simulink model "moteur_plus_gene_plus_charge_plus_frottement_22_09_2025"  (R2025b)
settings: Solver=VariableStepAuto  StartTime=0.0  StopTime=0.1  FixedStep=1e-4  RelTol=1e-3
values from neighbouring files (symbols this model uses):
  C0 = 2.4*10^-2    (= 0.024)    [donnee_moteur_seul_22_09_2025.m]
  f = (0.53*30*10^-2)/(1000*pi)    (= 5.06112719032e-05)    [donnee_moteur_seul_22_09_2025.m]
  J = 8.3e-5    (= 8.3e-05)    [donnee_moteur_seul_22_09_2025.m]
  Kphi = 0.127    [donnee_moteur_seul_22_09_2025.m]
  L = 2.2e-3    (= 0.0022)    [donnee_moteur_seul_22_09_2025.m]
  R = 1.52    [donnee_moteur_seul_22_09_2025.m]
  Rch = 10    [donnee_moteur_seul_22_09_2025.m]
  U = 48    [donnee_moteur_seul_22_09_2025.m]
settings Model: Creator=ltroullier01  LastModifiedBy=rudyv

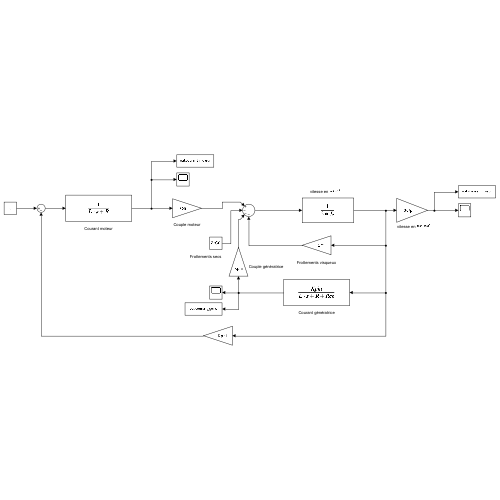
[thumbnail: Simulink's stored preview of the top-level diagram]
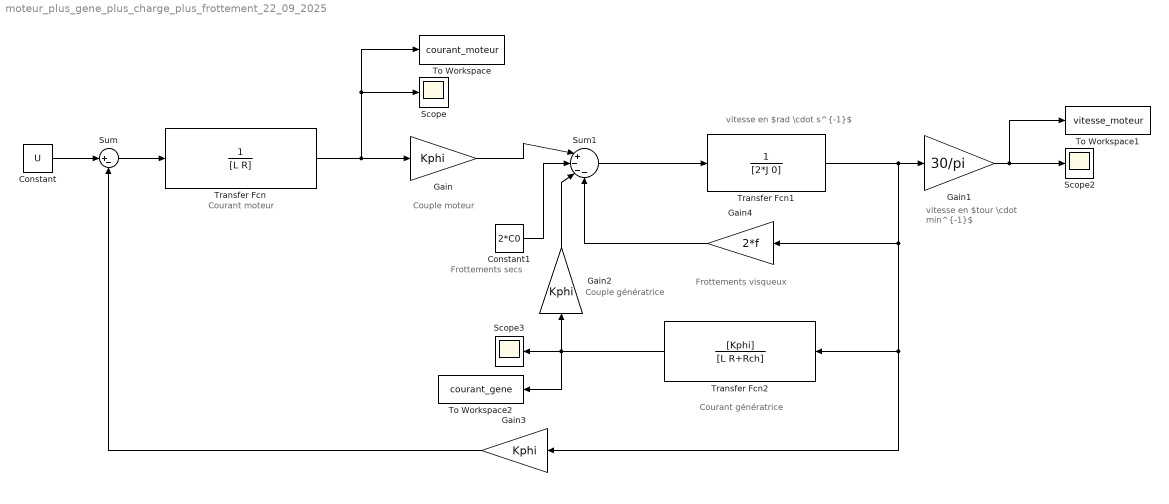
== system moteur_plus_gene_plus_charge_plus_frottement_22_09_2025 ==
  note: Courant génératrice
  note: Couple génératrice
  note: Frottements visqueux
  note: vitesse en $tour \cdot min^{-1}$
  note: Couple moteur
  note: Frottements secs
  note: Courant moteur
  note: vitesse en $rad \cdot s^{-1}$
  Constant : Constant  Value=U
  Constant1 : Constant  Value=2*C0
  Gain : Gain  Gain=Kphi
  Gain1 : Gain  Gain=30/pi
  Gain2 : Gain  Gain=Kphi
  Gain3 : Gain  Gain=Kphi
  Gain4 : Gain  Gain=2*f
  Scope : Scope
      settings: ActiveDisplayYMinimum=-4.9369832712561159  ActiveDisplayYMaximum=31.373841687864346
  Scope2 : Scope
      settings: ActiveDisplayYMinimum=-1903.7496929081253  ActiveDisplayYMaximum=5096.5030674299223  DataLoggingVariableName=ScopeData2
  Scope3 : Scope
      settings: ActiveDisplayYMinimum=-4.9369832712561159  ActiveDisplayYMaximum=31.373841687864346  DataLoggingVariableName=ScopeData3
  Sum : Sum  Inputs=|+-
  Sum1 : Sum  Inputs=|+---
  To Workspace : ToWorkspace  VariableName=courant_moteur  SaveFormat=Timeseries  SampleTime=-1
  To Workspace1 : ToWorkspace  VariableName=vitesse_moteur  SaveFormat=Timeseries  SampleTime=-1
  To Workspace2 : ToWorkspace  VariableName=courant_gene  SaveFormat=Timeseries  SampleTime=-1
  Transfer Fcn : TransferFcn  Denominator=[L R]
  Transfer Fcn1 : TransferFcn  Denominator=[2*J 0]
  Transfer Fcn2 : TransferFcn  Numerator=[Kphi]  Denominator=[L R+Rch]
  wires:
  Constant/1 -> Sum/1
  Sum/1 -> Transfer Fcn/1
  Transfer Fcn1/1 -> Gain1/1, Gain3/1, Transfer Fcn2/1, Gain4/1
  Gain1/1 -> To Workspace1/1, Scope2/1
  Transfer Fcn/1 -> To Workspace/1, Scope/1, Gain/1
  Gain/1 -> Sum1/1
  Sum1/1 -> Transfer Fcn1/1
  Transfer Fcn2/1 -> Gain2/1, Scope3/1, To Workspace2/1
  Gain3/1 -> Sum/2
  Gain2/1 -> Sum1/3
  Gain4/1 -> Sum1/4
  Constant1/1 -> Sum1/2
